simulink model "MECROKA_TWR_BLDC_01_main_model_v3_1"  (R2024a)
settings: Solver=ode23  StartTime=0.0  StopTime=25  RelTol=1e-3  EnableMultiTasking=on
model workspace (MATLAB code in the model file):
  | whl.rad = 0.045;
  | whl.thickness = 0.005;
  | 
  | tableWhl.contact.k = 1e4;
  | tableWhl.contact.b = 1e2;
  | tableWhl.velocity_threshold = 0.05;
  | table.length = 10;
  | table.thickness = 0.02;
  | 
  | initial.pitch = 1; % Degrees
  | initial.heigth_offset = table.thickness/2+0.002;
  | initial.heigth =-whl.rad-initial.heigth_offset;
  | 
  | ChassisCG.mass = 0.4;
  | ChassisCG.axle_distance = 0.04;
  | 
  | axle.IMU_distance = 0.04;
  | 
  | axle.length = 0.18;
  | axle.radius = 0.005;
  | axle.mass = 0.001;
  | 
  | num_pol_pairs = 7;
  | 
  | steel.density = 8000; %kg/m^3
  | 
  | start_pos.x = 0;
  | start_pos.y = -0.5;
undefined symbols (not defined in the file): X, Y, Z
libraries: sm_lib x22, nesl_utility x12, Contact_Forces_Lib x2, Parts_Lib x2
(part 2 of 2)

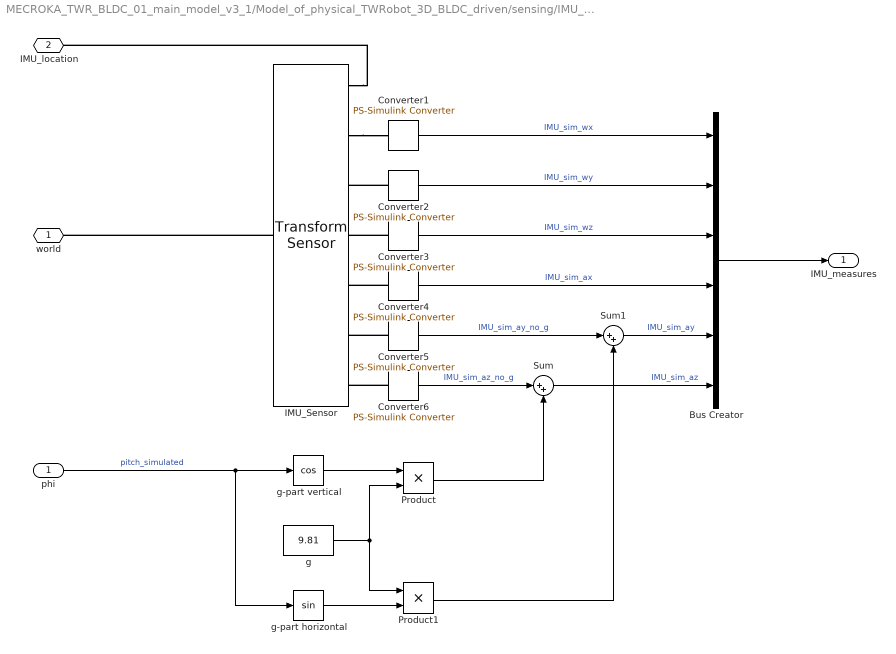
== system MECROKA_TWR_BLDC_01_main_model_v3_1/Model_of_physical_TWRobot_3D_BLDC_driven/sensing/IMU_model1 ==
  phi : Inport
  Bus Creator : BusCreator  Inputs=6
  Converter1 : nesl_utility/PS-Simulink Converter  PhysicalDomain=network_engine_domain  SubClassName=ps_output  LeftPortType=input  RightPortType=output  PseudoPeriodic=off  Frequencies=[]  VectorFormat=1-D array  Unit=rad/s  AffineConversion=off
  Converter2 : nesl_utility/PS-Simulink Converter  PhysicalDomain=network_engine_domain  SubClassName=ps_output  LeftPortType=input  RightPortType=output  PseudoPeriodic=off  Frequencies=[]  VectorFormat=1-D array  Unit=rad/s  AffineConversion=off
  Converter3 : nesl_utility/PS-Simulink Converter  PhysicalDomain=network_engine_domain  SubClassName=ps_output  LeftPortType=input  RightPortType=output  PseudoPeriodic=off  Frequencies=[]  VectorFormat=1-D array  Unit=rad/s  AffineConversion=off
  Converter4 : nesl_utility/PS-Simulink Converter  PhysicalDomain=network_engine_domain  SubClassName=ps_output  LeftPortType=input  RightPortType=output  PseudoPeriodic=off  Frequencies=[]  VectorFormat=1-D array  Unit=m/s^2  AffineConversion=off
  Converter5 : nesl_utility/PS-Simulink Converter  PhysicalDomain=network_engine_domain  SubClassName=ps_output  LeftPortType=input  RightPortType=output  PseudoPeriodic=off  Frequencies=[]  VectorFormat=1-D array  Unit=m/s^2  AffineConversion=off
  Converter6 : nesl_utility/PS-Simulink Converter  PhysicalDomain=network_engine_domain  SubClassName=ps_output  LeftPortType=input  RightPortType=output  PseudoPeriodic=off  Frequencies=[]  VectorFormat=1-D array  Unit=m/s^2  AffineConversion=off
  IMU_Sensor : sm_lib/Frames and Transforms/Transform Sensor  MeasurementFrame=NonRotatingFollower  RotationSequence=XYX  SenseAngle=off  SenseAxis=off  SenseQ=off  SenseR=off  SenseRotationSequence=off  SenseOmegaX=on  SenseOmegaY=on  SenseOmegaZ=on  SenseOmega=off  SenseQDot=off  SenseRDot=off  SenseRotationSequenceDot=off  SenseAlphaX=off  SenseAlphaY=off  SenseAlphaZ=off  SenseAlpha=off  SenseQDDot=off  SenseRDDot=off  SenseX=off  SenseY=off  SenseZ=off  SenseXYZ=off  SenseRad=off  SenseAzim=off  SenseDist=off  SenseInc=off  SenseXDot=off  SenseYDot=off  SenseZDot=off  SenseXYZDot=off  SenseRadDot=off  SenseAzimDot=off  SenseDistDot=off  SenseIncDot=off  SenseXDDot=on  SenseYDDot=on  SenseZDDot=on  SenseXYZDDot=off  SenseRadDDot=off  SenseAzimDDot=off  SenseDistDDot=off  SenseIncDDot=off
  Product : Product
  Product1 : Product
  Sum : Sum  Inputs=|++
  Sum1 : Sum  Inputs=|++
  g : Constant  Value=9.81
  g-part horizontal : Trigonometry
  g-part vertical : Trigonometry  Operator=cos
  world : PMIOPort  Side=Left
  IMU_location : PMIOPort  Port=2  Side=Left
  IMU_measures : Outport  VectorParamsAs1DForOutWhenUnconnected=off
  wires:
  Converter1/1 -> Bus Creator/1  "IMU_sim_wx"
  Converter2/1 -> Bus Creator/2  "IMU_sim_wy"
  Converter3/1 -> Bus Creator/3  "IMU_sim_wz"
  Converter4/1 -> Bus Creator/4  "IMU_sim_ax"
  Converter5/1 -> Sum1/1  "IMU_sim_ay_no_g"
  Converter6/1 -> Sum/1  "IMU_sim_az_no_g"
  Sum/1 -> Bus Creator/6  "IMU_sim_az"
  Sum1/1 -> Bus Creator/5  "IMU_sim_ay"
  phi/1 -> g-part horizontal/1, g-part vertical/1  "pitch_simulated"
  g-part vertical/1 -> Product/1
  g/1 -> Product/2, Product1/1
  Product/1 -> Sum/2
  g-part horizontal/1 -> Product1/2
  Product1/1 -> Sum1/2
  Bus Creator/1 -> IMU_measures/1
  connections:
  IMU_Sensor/LConn1 -- world/RConn1
  IMU_Sensor/RConn1 -- IMU_location/RConn1
  IMU_Sensor/RConn2 -- Converter1/LConn1
  Converter2/LConn1 -- IMU_Sensor/RConn3
  Converter3/LConn1 -- IMU_Sensor/RConn4
  Converter4/LConn1 -- IMU_Sensor/RConn5
  Converter5/LConn1 -- IMU_Sensor/RConn6
  Converter6/LConn1 -- IMU_Sensor/RConn7

== matlab function MECROKA_TWR_BLDC_01_main_model_v3_1/Model_of_physical_TWRobot_3D_BLDC_driven/sensing/MATLAB Function ==
  data: eulers input; pitchangle output
function pitchangle = euler2pitch(eulers)

pitchangle = atan2(eulers(3),eulers(6));

== matlab function MECROKA_TWR_BLDC_01_main_model_v3_1/phase voltages to BLDC motion conversion/MATLAB Function1 ==
  data: u input; u_last input; delta_phi output
function delta_phi  = fcn(u, u_last)
%#codegen

p1x = u(1)+u(2)*cos(2*pi/3)+u(3)*cos(4*pi/3);
p1y = u(2)*sin(2*pi/3)+u(3)*sin(4*pi/3);
p2x = u_last(1)+u_last(2)*cos(2*pi/3)+u_last(3)*cos(4*pi/3);
p2y = u_last(2)*sin(2*pi/3)+u_last(3)*sin(4*pi/3);
ph1 = atan2(p1y,p1x);
ph2 = atan2(p2y,p2x);
delta_phi = ph2-ph1;
if delta_phi < -pi/2;
    delta_phi = delta_phi+2*pi;
end
if delta_phi > pi/2;
        delta_phi = delta_phi-2*pi;
end

== matlab function MECROKA_TWR_BLDC_01_main_model_v3_1/phase voltages to BLDC motion conversion/MATLAB Function ==
  data: u input; u_last input; delta_phi output
function delta_phi  = fcn(u, u_last)
%#codegen

p1x = u(1)+u(2)*cos(2*pi/3)+u(3)*cos(4*pi/3);
p1y = u(2)*sin(2*pi/3)+u(3)*sin(4*pi/3);
p2x = u_last(1)+u_last(2)*cos(2*pi/3)+u_last(3)*cos(4*pi/3);
p2y = u_last(2)*sin(2*pi/3)+u_last(3)*sin(4*pi/3);
ph1 = atan2(p1y,p1x);
ph2 = atan2(p2y,p2x);
delta_phi = ph2-ph1;
if delta_phi < -pi/2;
    delta_phi = delta_phi+2*pi;
end
if delta_phi > pi/2;
        delta_phi = delta_phi-2*pi;
end
